simulink model "Lab1A_Task_2_3"  (R2019b)
settings: Solver=VariableStepAuto  StartTime=0.0  StopTime=10.0  RelTol=1e-3
settings Model: Creator=sinow  LastModifiedBy=sinow

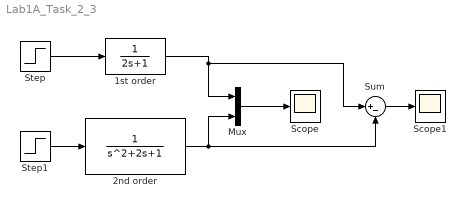
== system Lab1A_Task_2_3 ==
  1st order : TransferFcn  Denominator=[2 1]
  2nd order : TransferFcn
  Mux : Mux  Inputs=2
  Scope : Scope
  Scope1 : Scope
  Step : Step  Time=0  SampleTime=0
  Step1 : Step  Time=0  SampleTime=0
  Sum : Sum  Inputs=|+-
  wires:
  Step/1 -> 1st order/1
  Step1/1 -> 2nd order/1
  1st order/1 -> Sum/1, Mux/1
  2nd order/1 -> Sum/2, Mux/2
  Mux/1 -> Scope/1
  Sum/1 -> Scope1/1
